simulink model "model_zbiornik"  (R2018b)
settings: Solver=FixedStepAuto  StartTime=0.0  StopTime=100  FixedStep=0.01  RelTol=1e-3
values from neighbouring files (symbols this model uses):
  A = 0.06*0.07    (= 0.0042)    [definicja_parametrow_zbiornika.m]
  aa = pi*0.007*0.007    (= 0.000153938040026)    [definicja_parametrow_zbiornika.m]
  ab = pi*0.005*0.005    (= 7.85398163397e-05)    [definicja_parametrow_zbiornika.m]
  ac = pi*0.005*0.005    (= 7.85398163397e-05)    [definicja_parametrow_zbiornika.m]
  Ca = 1    [definicja_parametrow_zbiornika.m]
  Cb = 0.5    [definicja_parametrow_zbiornika.m]
  Cc = 0.5    [definicja_parametrow_zbiornika.m]
  gr = 9.81    [definicja_parametrow_zbiornika.m]
  kp = 7.3333*10^(-6)    (= 7.3333e-06)    [definicja_parametrow_zbiornika.m]
  Qmax = (4400*0.01*0.01*0.01)/60    (= 7.33333333333e-05)    [definicja_parametrow_zbiornika.m]
libraries: simulink x1
settings Model: Creator=Dominik  LastModifiedBy=user
settings DebuggingCC: LibraryContextMissingDiagnostic=none
settings SFSimCC: SimUseLocalCustomCode=off
settings RTWCC: RTWUseLocalCustomCode=off

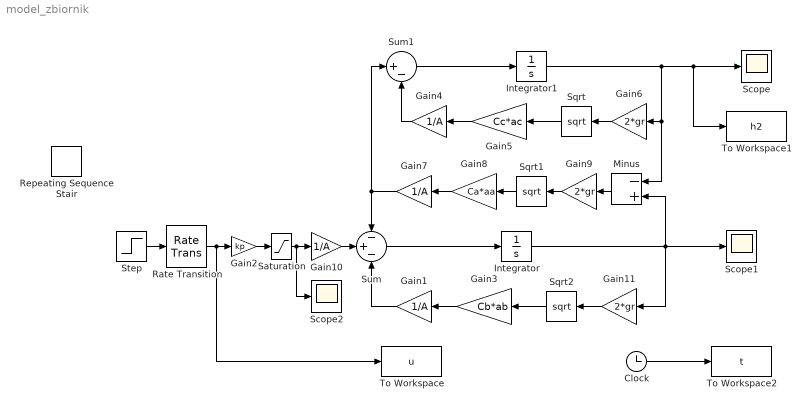
== system model_zbiornik ==
  Clock : Clock
  Gain{1,4,7,10} (4 alike) : Gain  Gain=1/A
  Gain11 : Gain  Gain=2*gr
  Gain2 : Gain  Gain=kp
  Gain3 : Gain  Gain=Cb*ab
  Gain5 : Gain  Gain=Cc*ac
  Gain6 : Gain  Gain=2*gr
  Gain8 : Gain  Gain=Ca*aa
  Gain9 : Gain  Gain=2*gr
  Integrator : Integrator  LimitOutput=on  LowerSaturationLimit=0
  Integrator1 : Integrator  LimitOutput=on  LowerSaturationLimit=0
  Minus : Sum  Inputs=-+
  Rate Transition : RateTransition
  Repeating Sequence Stair : simulink/Sources/Repeating Sequence Stair  OutValues="[6  7 2 4 1 1 1 2 2 2 2 4 12 33 22 11 9 3 4 2 2 2 2 2 2 2 4 4 4 4 4 1 1].'"  tsamp=3  OutMin=[]  OutMax=[]  OutDataTypeStr=double  OutputDataTypeScalingMode=double  OutDataType=fixdt(0,8)  ConRadixGroup=Best Precision: Vector-wise  OutScaling=2^-12
  Saturation : Saturate  UpperLimit=Qmax  LowerLimit=0
  Scope : Scope
  Scope1 : Scope
  Scope2 : Scope
  Sqrt : Sqrt  OutputSignalType=real  SaturateOnIntegerOverflow=on
  Sqrt1 : Sqrt  OutputSignalType=real  SaturateOnIntegerOverflow=on
  Sqrt2 : Sqrt  OutputSignalType=real  SaturateOnIntegerOverflow=on
  Step : Step  Time=4  After=10  SampleTime=0
  Sum : Sum  Inputs=-+-
  Sum1 : Sum  Inputs=|+-
  To Workspace : ToWorkspace  VariableName=u  SampleTime=-1
  To Workspace1 : ToWorkspace  VariableName=h2  SampleTime=-1
  To Workspace2 : ToWorkspace  VariableName=t  SampleTime=-1
  wires:
  Sum/1 -> Integrator/1
  Gain10/1 -> Sum/2
  Gain2/1 -> Saturation/1
  Clock/1 -> To Workspace2/1
  Integrator1/1 -> Minus/1, Gain6/1, To Workspace1/1, Scope/1
  Sum1/1 -> Integrator1/1
  Gain5/1 -> Gain4/1
  Gain6/1 -> Sqrt/1
  Gain4/1 -> Sum1/2
  Gain8/1 -> Gain7/1
  Sqrt1/1 -> Gain8/1
  Gain9/1 -> Sqrt1/1
  Minus/1 -> Gain9/1
  Gain7/1 -> Sum/1, Sum1/1
  Sqrt/1 -> Gain5/1
  Gain3/1 -> Gain1/1
  Gain11/1 -> Sqrt2/1
  Sqrt2/1 -> Gain3/1
  Gain1/1 -> Sum/3
  Integrator/1 -> Minus/2, Gain11/1, Scope1/1
  Step/1 -> Rate Transition/1
  Rate Transition/1 -> Gain2/1, To Workspace/1
  Saturation/1 -> Scope2/1, Gain10/1
